simulink model "mrefrobotarm_modified_previous_y_error_previous_u"  (R2018b)
settings: Solver=FixedStepAuto  StartTime=0.0  StopTime=60  RelTol=1e-3  AbsTol=1e-6
undefined symbols (not defined in the file or in its folder): now, sfunxy2, simin
libraries: neural x368, simulink x1
(part 7 of 10)

== system mrefrobotarm_modified_previous_y_error_previous_u/bad_2 /Layer 2/Delays 1 ==
  "p{2}" : Inport  PortDimensions=64
      mask Display: e = 0.06;c1 = [120 230 180]/255;c2 = ([120 230 180]+0)/(256+128);c3 = ([120 230 180]+128)/(256+128);patch([0 1 1 0],[0 0 1 1],c1);patch([0 1 1 1-e 1-e 0+e],[0 0 1 1-e 0+e 0+e],c2);patch([0 0 1 1-e 0+e 0+e],[0 1 1 1-e 1-e 0+e],c3);plot([0 1 1 0 0],[0 0 1 1 0]);
  mux : Mux  Inputs=1
      mask Display: e = 0.06;c1 = [120 150 230]/255;c2 = ([120 150 230]+0)/383;c3 = ([120 150 230]+128)/383;patch([0 1 1 0],[0 0 1 1],c1);patch([0 1 1 1-e 1-e 0+e],[0 0 1 1-e 0+e 0+e],c2);patch([0 0 1 1-e 0+e 0+e],[0 1 1 1-e 1-e 0+e],c3);plot([0 1 1 0 0],[0 0 1 1 0]);disp('Mux')
  "pd{2,1}" : Outport
      mask Display: e = 0.06;c1 = [120 230 180]/255;c2 = ([120 230 180]+0)/(256+128);c3 = ([120 230 180]+128)/(256+128);patch([0 1 1 0],[0 0 1 1],c1);patch([0 1 1 1-e 1-e 0+e],[0 0 1 1-e 0+e 0+e],c2);patch([0 0 1 1-e 0+e 0+e],[0 1 1 1-e 1-e 0+e],c3);plot([0 1 1 0 0],[0 0 1 1 0]);
  wires:
  "p{2}"/1 -> mux/1
  mux/1 -> "pd{2,1}"/1

== system mrefrobotarm_modified_previous_y_error_previous_u/bad_2 /Layer 2/LW{2,1} ==
  "ad{2,1}" : Inport  PortDimensions=64
      mask Display: e = 0.06;c1 = [120 230 180]/255;c2 = ([120 230 180]+0)/(256+128);c3 = ([120 230 180]+128)/(256+128);patch([0 1 1 0],[0 0 1 1],c1);patch([0 1 1 1-e 1-e 0+e],[0 0 1 1-e 0+e 0+e],c2);patch([0 0 1 1-e 0+e 0+e],[0 1 1 1-e 1-e 0+e],c3);plot([0 1 1 0 0],[0 0 1 1 0]);
  "IW{2,1}(1,:)'" : Constant  Value=[-0.234753869744093790483674411007086746394634246826171875;0.0626078209531036045110141685654525645077228546142578125;0.268385881292893480054573274173890240490436553955078125;0.0698142027739674098096855914263869635760784149169921875;-0.192488647302680060402479966796818189322948455810546875;-0.0220549078918776918223354499559718533419072628021240234375;0.07561329113330204909626530707100755535066127777099609375;-0.308099206445346940341778463334776461124420166015625;-1.6277000784937276645081283277249895036220550537109375;-0.1612353957030059625754603302993928082287311553955078125;-0.2220659402866968223921873004655935801565647125244140625;0.45574963928748435382232173651573248207569122314453125;-2.48258304572843702118234432418830692768096923828125;0.927785406087995756507780242827720940113067626953125;0.1674170074508223582387955730155226774513721466064453125;0.84281212940577387993101865504286251962184906005859375;1.90621775205526855501148020266555249691009521484375;1.647683116520871404730996800935827195644378662109375;1.339743047308181278509664480225183069705963134765625;-1.062702816025980379066595560288988053798675537109375;0.38403296644494744338516056814114563167095184326171875;-1.8781193450888438167822869218070991337299346923828125;-1.170853420079906559436722091049887239933013916015625;2.230101652600831929618152571492828428745269775390625;-0.511054155630024098400099319405853748321533203125;-0.63617663022596315780532449934980832040309906005859375;-0.2906927748343599571256845592870377004146575927734375;-0.5901018785507872177475974240223877131938934326171875;-0.8448699133245070047593117124051786959171295166015625;1.877979245622388049241635599173605442047119140625;-1.17923641706391446604129669140093028545379638671875;-1.09205020113977724349751952104270458221435546875;0.1657716248453909579918530425857170484960079193115234375;3.177274361730112683943616502801887691020965576171875;3.0036182706847966983332298696041107177734375;0.1091758551043676417346972584709874354302883148193359375;-3.1944235360597144079974896158091723918914794921875;0.05450977025433319245184549117766437120735645294189453125;-1.7024350481800485379579868094879202544689178466796875;-0.6752862890832960207632140736677683889865875244140625;-0.11995561605138908845002987391126225702464580535888671875;-1.745747931820843756867134288768284022808074951171875;0.201795588848985907315380927684600464999675750732421875;1.07301675002311913686980915372259914875030517578125;-0.492892609782685564567827896098606288433074951171875;-0.494936550864729429832777896081097424030303955078125;1.8537384597422918997011720421141944825649261474609375;-0.5342149981282282578121112237568013370037078857421875;-0.882464218867245353550288200494833290576934814453125;-0.759907231887786860369260466541163623332977294921875;0.5978789092341834088273344605113379657268524169921875;-1.0750175619194204390538516236119903624057769775390625;-0.476446367359680655884091038387850858271121978759765625;0.79687849589455728160913849933422170579433441162109375;-0.2492235434928220250139219160701031796634197235107421875;0.3278655352152355373362979662488214671611785888671875;0.1720686516033732849084714189302758313715457916259765625;0.06941560089039659764420520104977185837924480438232421875;-0.63969497582223155962566352172871120274066925048828125;-0.0743124451882172520900127210552454926073551177978515625;-0.0258588106974563212980822157760485424660146236419677734375;-0.410054324959951532747481905971653759479522705078125;0.309660024662619048907430396866402588784694671630859375;0.1493281175622258316604273886696319095790386199951171875]
      mask Display: e = 0.06;c1 = [120 150 230]/255;c2 = ([120 150 230]+0)/383;c3 = ([120 150 230]+128)/383;patch([0 1 1 0],[0 0 1 1],c1);patch([0 1 1 1-e 1-e 0+e],[0 0 1 1-e 0+e 0+e],c2);patch([0 0 1 1-e 0+e 0+e],[0 1 1 1-e 1-e 0+e],c3);plot([0 1 1 0 0],[0 0 1 1 0]);disp('weights');
  Mux : Mux  Inputs=1
      mask Display: e = 0.06;c1 = [120 150 230]/255;c2 = ([120 150 230]+0)/383;c3 = ([120 150 230]+128)/383;patch([0 1 1 0],[0 0 1 1],c1);patch([0 1 1 1-e 1-e 0+e],[0 0 1 1-e 0+e 0+e],c2);patch([0 0 1 1-e 0+e 0+e],[0 1 1 1-e 1-e 0+e],c3);plot([0 1 1 0 0],[0 0 1 1 0]);disp('Mux');
  dotprod1 : neural/Weight Functions/dotprod
  "lz{2,1}" : Outport
      mask Display: e = 0.06;c1 = [120 230 180]/255;c2 = ([120 230 180]+0)/(256+128);c3 = ([120 230 180]+128)/(256+128);patch([0 1 1 0],[0 0 1 1],c1);patch([0 1 1 1-e 1-e 0+e],[0 0 1 1-e 0+e 0+e],c2);patch([0 0 1 1-e 0+e 0+e],[0 1 1 1-e 1-e 0+e],c3);plot([0 1 1 0 0],[0 0 1 1 0]);
  wires:
  "IW{2,1}(1,:)'"/1 -> dotprod1/1
  "ad{2,1}"/1 -> dotprod1/2
  dotprod1/1 -> Mux/1
  Mux/1 -> "lz{2,1}"/1

== system mrefrobotarm_modified_previous_y_error_previous_u/big_bad/Layer 1/Delays 1 ==
  "p{1}" : Inport  PortDimensions=7
      mask Display: e = 0.06;c1 = [120 230 180]/255;c2 = ([120 230 180]+0)/(256+128);c3 = ([120 230 180]+128)/(256+128);patch([0 1 1 0],[0 0 1 1],c1);patch([0 1 1 1-e 1-e 0+e],[0 0 1 1-e 0+e 0+e],c2);patch([0 0 1 1-e 0+e 0+e],[0 1 1 1-e 1-e 0+e],c3);plot([0 1 1 0 0],[0 0 1 1 0]);
  mux : Mux  Inputs=1
      mask Display: e = 0.06;c1 = [120 150 230]/255;c2 = ([120 150 230]+0)/383;c3 = ([120 150 230]+128)/383;patch([0 1 1 0],[0 0 1 1],c1);patch([0 1 1 1-e 1-e 0+e],[0 0 1 1-e 0+e 0+e],c2);patch([0 0 1 1-e 0+e 0+e],[0 1 1 1-e 1-e 0+e],c3);plot([0 1 1 0 0],[0 0 1 1 0]);disp('Mux')
  "pd{1,1}" : Outport
      mask Display: e = 0.06;c1 = [120 230 180]/255;c2 = ([120 230 180]+0)/(256+128);c3 = ([120 230 180]+128)/(256+128);patch([0 1 1 0],[0 0 1 1],c1);patch([0 1 1 1-e 1-e 0+e],[0 0 1 1-e 0+e 0+e],c2);patch([0 0 1 1-e 0+e 0+e],[0 1 1 1-e 1-e 0+e],c3);plot([0 1 1 0 0],[0 0 1 1 0]);
  wires:
  "p{1}"/1 -> mux/1
  mux/1 -> "pd{1,1}"/1

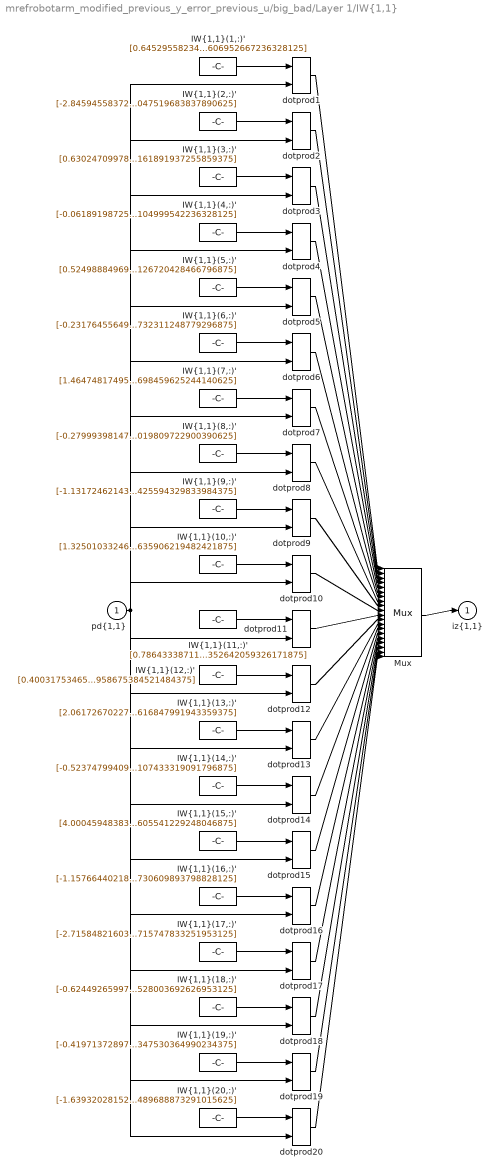
== system mrefrobotarm_modified_previous_y_error_previous_u/big_bad/Layer 1/IW{1,1} ==
  "pd{1,1}" : Inport  PortDimensions=7
      mask Display: e = 0.06;c1 = [120 230 180]/255;c2 = ([120 230 180]+0)/(256+128);c3 = ([120 230 180]+128)/(256+128);patch([0 1 1 0],[0 0 1 1],c1);patch([0 1 1 1-e 1-e 0+e],[0 0 1 1-e 0+e 0+e],c2);patch([0 0 1 1-e 0+e 0+e],[0 1 1 1-e 1-e 0+e],c3);plot([0 1 1 0 0],[0 0 1 1 0]);
  "IW{1,1}(1,:)'" : Constant  Value=[0.64529558234887385292921635482343845069408416748046875;-0.1945897902722976413603106493610539473593235015869140625;0.59349829296596279260000983413192443549633026123046875;-1.6122567894332207050211991372634656727313995361328125;-0.416808711676973697723980194496107287704944610595703125;-0.11079987642376055989590355466134496964514255523681640625;0.332085522631030471973900830562342889606952667236328125]
      mask Display: e = 0.06;c1 = [120 150 230]/255;c2 = ([120 150 230]+0)/383;c3 = ([120 150 230]+128)/383;patch([0 1 1 0],[0 0 1 1],c1);patch([0 1 1 1-e 1-e 0+e],[0 0 1 1-e 0+e 0+e],c2);patch([0 0 1 1-e 0+e 0+e],[0 1 1 1-e 1-e 0+e],c3);plot([0 1 1 0 0],[0 0 1 1 0]);disp('Weights');
  "IW{1,1}(10,:)'" : Constant  Value=[1.3250103324626432144128784784697927534580230712890625;-1.7914401294432831246439263850334100425243377685546875;0.336675918691728137677188215093337930738925933837890625;0.19229875400490159531585732111125253140926361083984375;1.225747968501573748056898693903349339962005615234375;-0.83402516067975251967681060705217532813549041748046875;-0.82008817609693884786992157387430779635906219482421875]
      mask Display: e = 0.06;c1 = [120 150 230]/255;c2 = ([120 150 230]+0)/383;c3 = ([120 150 230]+128)/383;patch([0 1 1 0],[0 0 1 1],c1);patch([0 1 1 1-e 1-e 0+e],[0 0 1 1-e 0+e 0+e],c2);patch([0 0 1 1-e 0+e 0+e],[0 1 1 1-e 1-e 0+e],c3);plot([0 1 1 0 0],[0 0 1 1 0]);disp('Weights');
  "IW{1,1}(11,:)'" : Constant  Value=[0.78643338711871713098133795938338153064250946044921875;-0.91869007485024367642978404546738602221012115478515625;-0.4593294706246362490986712145968340337276458740234375;-0.493554536494603457441598948207683861255645751953125;2.08831224755974798057422958663664758205413818359375;1.020857334988159781374861267977394163608551025390625;-0.80911613686495698072320692517678253352642059326171875]
      mask Display: e = 0.06;c1 = [120 150 230]/255;c2 = ([120 150 230]+0)/383;c3 = ([120 150 230]+128)/383;patch([0 1 1 0],[0 0 1 1],c1);patch([0 1 1 1-e 1-e 0+e],[0 0 1 1-e 0+e 0+e],c2);patch([0 0 1 1-e 0+e 0+e],[0 1 1 1-e 1-e 0+e],c3);plot([0 1 1 0 0],[0 0 1 1 0]);disp('Weights');
  "IW{1,1}(12,:)'" : Constant  Value=[0.400317534652308515408236644361750222742557525634765625;1.211389184468974367092641841736622154712677001953125;-0.389719995331499313717671384438290260732173919677734375;-1.2662597452397010844293845366337336599826812744140625;-1.6284049834295741820966441082418896257877349853515625;-0.21922229581120566965779516976908780634403228759765625;-1.5793703622594266189338441108702681958675384521484375]
      mask Display: e = 0.06;c1 = [120 150 230]/255;c2 = ([120 150 230]+0)/383;c3 = ([120 150 230]+128)/383;patch([0 1 1 0],[0 0 1 1],c1);patch([0 1 1 1-e 1-e 0+e],[0 0 1 1-e 0+e 0+e],c2);patch([0 0 1 1-e 0+e 0+e],[0 1 1 1-e 1-e 0+e],c3);plot([0 1 1 0 0],[0 0 1 1 0]);disp('Weights');
  "IW{1,1}(13,:)'" : Constant  Value=[2.06172670227497345507572390488348901271820068359375;-1.6312697749777440581198106883675791323184967041015625;-0.10866045476962458982139736463068402372300624847412109375;0.67503853769883104263271889067254960536956787109375;0.05493398925839632074286100760218687355518341064453125;-1.2986214924140000448460341431200504302978515625;0.492688647336579632618480673045269213616847991943359375]
      mask Display: e = 0.06;c1 = [120 150 230]/255;c2 = ([120 150 230]+0)/383;c3 = ([120 150 230]+128)/383;patch([0 1 1 0],[0 0 1 1],c1);patch([0 1 1 1-e 1-e 0+e],[0 0 1 1-e 0+e 0+e],c2);patch([0 0 1 1-e 0+e 0+e],[0 1 1 1-e 1-e 0+e],c3);plot([0 1 1 0 0],[0 0 1 1 0]);disp('Weights');
  "IW{1,1}(14,:)'" : Constant  Value=[-0.523747994099180491645029178471304476261138916015625;-1.047233970140400316495288279838860034942626953125;-1.1102699039564780658650988698354922235012054443359375;-0.5702346662702872936989706431631930172443389892578125;-0.354033765235858666198254240953247062861919403076171875;-0.2081790845373985010535733408687519840896129608154296875;1.09831668607501153900329882162623107433319091796875]
      mask Display: e = 0.06;c1 = [120 150 230]/255;c2 = ([120 150 230]+0)/383;c3 = ([120 150 230]+128)/383;patch([0 1 1 0],[0 0 1 1],c1);patch([0 1 1 1-e 1-e 0+e],[0 0 1 1-e 0+e 0+e],c2);patch([0 0 1 1-e 0+e 0+e],[0 1 1 1-e 1-e 0+e],c3);plot([0 1 1 0 0],[0 0 1 1 0]);disp('Weights');
  "IW{1,1}(15,:)'" : Constant  Value=[4.00045948383238414436391394701786339282989501953125;-1.7593207792483323004262274480424821376800537109375;-1.8464283444473832407339841665816493332386016845703125;-0.12316972502595584237905512736688251607120037078857421875;-1.5623289864460219167341392676462419331073760986328125;-2.01311459638506651259604041115380823612213134765625;-0.8521233205842999591794750813278369605541229248046875]
      mask Display: e = 0.06;c1 = [120 150 230]/255;c2 = ([120 150 230]+0)/383;c3 = ([120 150 230]+128)/383;patch([0 1 1 0],[0 0 1 1],c1);patch([0 1 1 1-e 1-e 0+e],[0 0 1 1-e 0+e 0+e],c2);patch([0 0 1 1-e 0+e 0+e],[0 1 1 1-e 1-e 0+e],c3);plot([0 1 1 0 0],[0 0 1 1 0]);disp('Weights');
  "IW{1,1}(16,:)'" : Constant  Value=[-1.1576644021839952447550103897810913622379302978515625;-1.0657958148743686965786992004723288118839263916015625;-0.95029258214202794174951804961892776191234588623046875;0.8926485091304263708167354707256890833377838134765625;0.64197334810276618366486900413292460143566131591796875;-1.6230328945070819912643855786882340908050537109375;-1.08954214162409801502917616744525730609893798828125]
      mask Display: e = 0.06;c1 = [120 150 230]/255;c2 = ([120 150 230]+0)/383;c3 = ([120 150 230]+128)/383;patch([0 1 1 0],[0 0 1 1],c1);patch([0 1 1 1-e 1-e 0+e],[0 0 1 1-e 0+e 0+e],c2);patch([0 0 1 1-e 0+e 0+e],[0 1 1 1-e 1-e 0+e],c3);plot([0 1 1 0 0],[0 0 1 1 0]);disp('Weights');
  "IW{1,1}(17,:)'" : Constant  Value=[-2.715848216035800621881435290561057627201080322265625;3.54852805111261826453983303508721292018890380859375;1.0314188420478422880677271677996031939983367919921875;-1.7861596640978998351556583656929433345794677734375;-1.1440403115366140074371514856466092169284820556640625;-2.316622230946209892721299183904193341732025146484375;-1.0788987317369251872634094979730434715747833251953125]
      mask Display: e = 0.06;c1 = [120 150 230]/255;c2 = ([120 150 230]+0)/383;c3 = ([120 150 230]+128)/383;patch([0 1 1 0],[0 0 1 1],c1);patch([0 1 1 1-e 1-e 0+e],[0 0 1 1-e 0+e 0+e],c2);patch([0 0 1 1-e 0+e 0+e],[0 1 1 1-e 1-e 0+e],c3);plot([0 1 1 0 0],[0 0 1 1 0]);disp('Weights');
  "IW{1,1}(18,:)'" : Constant  Value=[-0.62449265997037339825936896886560134589672088623046875;1.3458495913616232986242948754807002842426300048828125;-0.96646654372549190004093588868272490799427032470703125;0.63618734494530304601767056738026440143585205078125;-0.487974232437826227481991736567579209804534912109375;-1.117999282768670443743985742912627756595611572265625;-0.59470875456635330369437042463687248528003692626953125]
      mask Display: e = 0.06;c1 = [120 150 230]/255;c2 = ([120 150 230]+0)/383;c3 = ([120 150 230]+128)/383;patch([0 1 1 0],[0 0 1 1],c1);patch([0 1 1 1-e 1-e 0+e],[0 0 1 1-e 0+e 0+e],c2);patch([0 0 1 1-e 0+e 0+e],[0 1 1 1-e 1-e 0+e],c3);plot([0 1 1 0 0],[0 0 1 1 0]);disp('Weights');
  "IW{1,1}(19,:)'" : Constant  Value=[-0.419713728971699617797952441833331249654293060302734375;0.72621640951271293484836633069789968430995941162109375;0.414880191996511771268529855660744942724704742431640625;0.2390452725663312349979605642147362232208251953125;-0.2075502420258710234435284291976131498813629150390625;-0.65808722407428488221370344035676680505275726318359375;-0.445916251008992625681770505252643488347530364990234375]
      mask Display: e = 0.06;c1 = [120 150 230]/255;c2 = ([120 150 230]+0)/383;c3 = ([120 150 230]+128)/383;patch([0 1 1 0],[0 0 1 1],c1);patch([0 1 1 1-e 1-e 0+e],[0 0 1 1-e 0+e 0+e],c2);patch([0 0 1 1-e 0+e 0+e],[0 1 1 1-e 1-e 0+e],c3);plot([0 1 1 0 0],[0 0 1 1 0]);disp('Weights');
  "IW{1,1}(2,:)'" : Constant  Value=[-2.8459455837235712039046120480634272098541259765625;0.1585791674640530113382652643849723972380161285400390625;0.59196721877598956762511761553469114005565643310546875;0.29334396882843816189989638587576337158679962158203125;2.092473411913708947196255394374020397663116455078125;2.2187164670997123749884849530644714832305908203125;0.536972066296338201851767735206522047519683837890625]
      mask Display: e = 0.06;c1 = [120 150 230]/255;c2 = ([120 150 230]+0)/383;c3 = ([120 150 230]+128)/383;patch([0 1 1 0],[0 0 1 1],c1);patch([0 1 1 1-e 1-e 0+e],[0 0 1 1-e 0+e 0+e],c2);patch([0 0 1 1-e 0+e 0+e],[0 1 1 1-e 1-e 0+e],c3);plot([0 1 1 0 0],[0 0 1 1 0]);disp('Weights');
  "IW{1,1}(20,:)'" : Constant  Value=[-1.639320281525530109689725577482022345066070556640625;-0.76559503756869684565344869042746722698211669921875;1.3513927864564438952044156394549645483493804931640625;-0.275669130171111886884460773217142559587955474853515625;0.196701462748026079108143449047929607331752777099609375;0.1577383287839831116361466456510243006050586700439453125;-0.19406100382370594648051564945490099489688873291015625]
      mask Display: e = 0.06;c1 = [120 150 230]/255;c2 = ([120 150 230]+0)/383;c3 = ([120 150 230]+128)/383;patch([0 1 1 0],[0 0 1 1],c1);patch([0 1 1 1-e 1-e 0+e],[0 0 1 1-e 0+e 0+e],c2);patch([0 0 1 1-e 0+e 0+e],[0 1 1 1-e 1-e 0+e],c3);plot([0 1 1 0 0],[0 0 1 1 0]);disp('Weights');
  "IW{1,1}(3,:)'" : Constant  Value=[0.630247099788600717573672227445058524608612060546875;1.5900953333789040744505882685189135372638702392578125;-0.89669287951352549814743042588816024363040924072265625;0.59962114718742920427274611938628368079662322998046875;0.84926285805418022523127774547901935875415802001953125;0.0118635669976363371247440881006696145050227642059326171875;-1.05202565288192939618738819262944161891937255859375]
      mask Display: e = 0.06;c1 = [120 150 230]/255;c2 = ([120 150 230]+0)/383;c3 = ([120 150 230]+128)/383;patch([0 1 1 0],[0 0 1 1],c1);patch([0 1 1 1-e 1-e 0+e],[0 0 1 1-e 0+e 0+e],c2);patch([0 0 1 1-e 0+e 0+e],[0 1 1 1-e 1-e 0+e],c3);plot([0 1 1 0 0],[0 0 1 1 0]);disp('Weights');
  "IW{1,1}(4,:)'" : Constant  Value=[-0.061891987255859197414320505004070582799613475799560546875;0.5219779411656577661204892137902788817882537841796875;0.70843583939288079509566387059749104082584381103515625;-1.5121436342542808883848692858009599149227142333984375;-0.162512764221157290922548099842970259487628936767578125;-0.68634292134649055316941712590050883591175079345703125;-0.59174741102794314873136727328528650104999542236328125]
      mask Display: e = 0.06;c1 = [120 150 230]/255;c2 = ([120 150 230]+0)/383;c3 = ([120 150 230]+128)/383;patch([0 1 1 0],[0 0 1 1],c1);patch([0 1 1 1-e 1-e 0+e],[0 0 1 1-e 0+e 0+e],c2);patch([0 0 1 1-e 0+e 0+e],[0 1 1 1-e 1-e 0+e],c3);plot([0 1 1 0 0],[0 0 1 1 0]);disp('Weights');
  "IW{1,1}(5,:)'" : Constant  Value=[0.5249888496989048025653801232692785561084747314453125;0.1811788365727916294556365528478636406362056732177734375;-0.0706982962558852789936025828865240328013896942138671875;0.76054708611638532911314314333139918744564056396484375;-0.062040258638566152249449459077368373982608318328857421875;0.98696901394403846463632135055377148091793060302734375;1.034339583684487973158638851600699126720428466796875]
      mask Display: e = 0.06;c1 = [120 150 230]/255;c2 = ([120 150 230]+0)/383;c3 = ([120 150 230]+128)/383;patch([0 1 1 0],[0 0 1 1],c1);patch([0 1 1 1-e 1-e 0+e],[0 0 1 1-e 0+e 0+e],c2);patch([0 0 1 1-e 0+e 0+e],[0 1 1 1-e 1-e 0+e],c3);plot([0 1 1 0 0],[0 0 1 1 0]);disp('Weights');
  "IW{1,1}(6,:)'" : Constant  Value=[-0.23176455649559013494354076101444661617279052734375;1.61825927500757327237579374923370778560638427734375;-0.00050171377653901948721892889437867779633961617946624755859375;-0.7477355096421127722550181715632788836956024169921875;2.36800807384332046012787031941115856170654296875;-0.2326701825135666645838483646002714522182941436767578125;-0.52951977817398787617975131070124916732311248779296875]
      mask Display: e = 0.06;c1 = [120 150 230]/255;c2 = ([120 150 230]+0)/383;c3 = ([120 150 230]+128)/383;patch([0 1 1 0],[0 0 1 1],c1);patch([0 1 1 1-e 1-e 0+e],[0 0 1 1-e 0+e 0+e],c2);patch([0 0 1 1-e 0+e 0+e],[0 1 1 1-e 1-e 0+e],c3);plot([0 1 1 0 0],[0 0 1 1 0]);disp('Weights');
  "IW{1,1}(7,:)'" : Constant  Value=[1.4647481749561104269474753891699947416782379150390625;-1.48930980763576759073885114048607647418975830078125;-0.211199358264218706171533312954124994575977325439453125;-0.2003059822065408057678581599247991107404232025146484375;-1.40474454751325783519178003189153969287872314453125;1.894054731069508168417314664111472666263580322265625;0.51576699938655468091752709369757212698459625244140625]
      mask Display: e = 0.06;c1 = [120 150 230]/255;c2 = ([120 150 230]+0)/383;c3 = ([120 150 230]+128)/383;patch([0 1 1 0],[0 0 1 1],c1);patch([0 1 1 1-e 1-e 0+e],[0 0 1 1-e 0+e 0+e],c2);patch([0 0 1 1-e 0+e 0+e],[0 1 1 1-e 1-e 0+e],c3);plot([0 1 1 0 0],[0 0 1 1 0]);disp('Weights');
  "IW{1,1}(8,:)'" : Constant  Value=[-0.279993981474716824298099027146236039698123931884765625;-1.3388618528925813055963089936994947493076324462890625;-0.45660369009358403591392061571241356432437896728515625;1.782573206194468351526438709697686135768890380859375;3.19766398279266983450952466228045523166656494140625;4.10357231567076308209607304888777434825897216796875;1.1503085187380401865908652325742878019809722900390625]
      mask Display: e = 0.06;c1 = [120 150 230]/255;c2 = ([120 150 230]+0)/383;c3 = ([120 150 230]+128)/383;patch([0 1 1 0],[0 0 1 1],c1);patch([0 1 1 1-e 1-e 0+e],[0 0 1 1-e 0+e 0+e],c2);patch([0 0 1 1-e 0+e 0+e],[0 1 1 1-e 1-e 0+e],c3);plot([0 1 1 0 0],[0 0 1 1 0]);disp('Weights');
  "IW{1,1}(9,:)'" : Constant  Value=[-1.1317246214326017739182361765415407717227935791015625;-0.33822557123675200951851138597703538835048675537109375;-0.2855194012811612669366923000779934227466583251953125;-1.061181656540413964506797128706239163875579833984375;-0.51307906959430338300620633162907324731349945068359375;0.8842064298724461313128131223493255674839019775390625;0.26611018560909283081628018408082425594329833984375]
      mask Display: e = 0.06;c1 = [120 150 230]/255;c2 = ([120 150 230]+0)/383;c3 = ([120 150 230]+128)/383;patch([0 1 1 0],[0 0 1 1],c1);patch([0 1 1 1-e 1-e 0+e],[0 0 1 1-e 0+e 0+e],c2);patch([0 0 1 1-e 0+e 0+e],[0 1 1 1-e 1-e 0+e],c3);plot([0 1 1 0 0],[0 0 1 1 0]);disp('Weights');
  Mux : Mux  Inputs=20
      mask Display: e = 0.06;c1 = [120 150 230]/255;c2 = ([120 150 230]+0)/383;c3 = ([120 150 230]+128)/383;patch([0 1 1 0],[0 0 1 1],c1);patch([0 1 1 1-e 1-e 0+e],[0 0 1 1-e 0+e 0+e],c2);patch([0 0 1 1-e 0+e 0+e],[0 1 1 1-e 1-e 0+e],c3);plot([0 1 1 0 0],[0 0 1 1 0]);disp('Mux');
  dotprod{1..20} (20 alike) : neural/Weight Functions/dotprod
  "iz{1,1}" : Outport
      mask Display: e = 0.06;c1 = [120 230 180]/255;c2 = ([120 230 180]+0)/(256+128);c3 = ([120 230 180]+128)/(256+128);patch([0 1 1 0],[0 0 1 1],c1);patch([0 1 1 1-e 1-e 0+e],[0 0 1 1-e 0+e 0+e],c2);patch([0 0 1 1-e 0+e 0+e],[0 1 1 1-e 1-e 0+e],c3);plot([0 1 1 0 0],[0 0 1 1 0]);
  wires:
  "IW{1,1}(1,:)'"/1 -> dotprod1/1
  "pd{1,1}"/1 -> dotprod1/2, dotprod2/2, dotprod3/2, dotprod4/2, dotprod5/2, dotprod6/2, dotprod7/2, dotprod8/2, dotprod9/2, dotprod10/2, dotprod11/2, dotprod12/2, dotprod13/2, dotprod14/2, dotprod15/2, dotprod16/2, dotprod17/2, dotprod18/2, dotprod19/2, dotprod20/2
  dotprod1/1 -> Mux/1
  "IW{1,1}(2,:)'"/1 -> dotprod2/1
  dotprod2/1 -> Mux/2
  "IW{1,1}(3,:)'"/1 -> dotprod3/1
  dotprod3/1 -> Mux/3
  "IW{1,1}(4,:)'"/1 -> dotprod4/1
  dotprod4/1 -> Mux/4
  "IW{1,1}(5,:)'"/1 -> dotprod5/1
  dotprod5/1 -> Mux/5
  "IW{1,1}(6,:)'"/1 -> dotprod6/1
  dotprod6/1 -> Mux/6
  "IW{1,1}(7,:)'"/1 -> dotprod7/1
  dotprod7/1 -> Mux/7
  "IW{1,1}(8,:)'"/1 -> dotprod8/1
  dotprod8/1 -> Mux/8
  "IW{1,1}(9,:)'"/1 -> dotprod9/1
  dotprod9/1 -> Mux/9
  "IW{1,1}(10,:)'"/1 -> dotprod10/1
  dotprod10/1 -> Mux/10
  "IW{1,1}(11,:)'"/1 -> dotprod11/1
  dotprod11/1 -> Mux/11
  "IW{1,1}(12,:)'"/1 -> dotprod12/1
  dotprod12/1 -> Mux/12
  "IW{1,1}(13,:)'"/1 -> dotprod13/1
  dotprod13/1 -> Mux/13
  "IW{1,1}(14,:)'"/1 -> dotprod14/1
  dotprod14/1 -> Mux/14
  "IW{1,1}(15,:)'"/1 -> dotprod15/1
  dotprod15/1 -> Mux/15
  "IW{1,1}(16,:)'"/1 -> dotprod16/1
  dotprod16/1 -> Mux/16
  "IW{1,1}(17,:)'"/1 -> dotprod17/1
  dotprod17/1 -> Mux/17
  "IW{1,1}(18,:)'"/1 -> dotprod18/1
  dotprod18/1 -> Mux/18
  "IW{1,1}(19,:)'"/1 -> dotprod19/1
  dotprod19/1 -> Mux/19
  "IW{1,1}(20,:)'"/1 -> dotprod20/1
  dotprod20/1 -> Mux/20
  Mux/1 -> "iz{1,1}"/1

== system mrefrobotarm_modified_previous_y_error_previous_u/big_bad/Layer 2/Delays 1 ==
  "p{2}" : Inport  PortDimensions=20
      mask Display: e = 0.06;c1 = [120 230 180]/255;c2 = ([120 230 180]+0)/(256+128);c3 = ([120 230 180]+128)/(256+128);patch([0 1 1 0],[0 0 1 1],c1);patch([0 1 1 1-e 1-e 0+e],[0 0 1 1-e 0+e 0+e],c2);patch([0 0 1 1-e 0+e 0+e],[0 1 1 1-e 1-e 0+e],c3);plot([0 1 1 0 0],[0 0 1 1 0]);
  mux : Mux  Inputs=1
      mask Display: e = 0.06;c1 = [120 150 230]/255;c2 = ([120 150 230]+0)/383;c3 = ([120 150 230]+128)/383;patch([0 1 1 0],[0 0 1 1],c1);patch([0 1 1 1-e 1-e 0+e],[0 0 1 1-e 0+e 0+e],c2);patch([0 0 1 1-e 0+e 0+e],[0 1 1 1-e 1-e 0+e],c3);plot([0 1 1 0 0],[0 0 1 1 0]);disp('Mux')
  "pd{2,1}" : Outport
      mask Display: e = 0.06;c1 = [120 230 180]/255;c2 = ([120 230 180]+0)/(256+128);c3 = ([120 230 180]+128)/(256+128);patch([0 1 1 0],[0 0 1 1],c1);patch([0 1 1 1-e 1-e 0+e],[0 0 1 1-e 0+e 0+e],c2);patch([0 0 1 1-e 0+e 0+e],[0 1 1 1-e 1-e 0+e],c3);plot([0 1 1 0 0],[0 0 1 1 0]);
  wires:
  "p{2}"/1 -> mux/1
  mux/1 -> "pd{2,1}"/1
